simulink model "sl_EstimacDinamic"  (Simulink 9.1)
settings: Solver=ode45  StartTime=0.0  StopTime=40  RelTol=1e-8  EnableMultiTasking=on
values from neighbouring files (symbols this model uses):
  Aa_1 = Aa_1/50    (= 0.004)    [DatosSimAcDir_Exp.m]    (also in DatosSimSenoides.m = 1; DatosSimSenoides_Exp.m = 2)
  Aa_2 = Aa_2/30    (= 6.66666666667)    [DatosSimAcDir_Exp.m]    (also in DatosSimSenoides.m = 1; DatosSimSenoides_Exp.m = 0.5)
  Aa_3 = Aa_3/15    (= 0.266666666667)    [DatosSimAcDir_Exp.m]    (also in DatosSimSenoides.m = 5; DatosSimSenoides_Exp.m = 0.5)
  Ab_1 = Ab_1/50    (= 6e-05)    [DatosSimAcDir_Exp.m]    (also in DatosSimSenoides.m = 2; DatosSimSenoides_Exp.m = 3)
  Ab_3 = Ab_3/15    (= 1)    [DatosSimAcDir_Exp.m]    (also in DatosSimSenoides.m = 6; DatosSimSenoides_Exp.m = 2)
  Im_cc1 = Im_cc1/50    (= 0)    [DatosSimAcDir_Exp.m]    (also in DatosSimSenoides.m; DatosSimSenoides_Exp.m)
  Im_cc2 = Im_cc2/30    (= 96.6666666667)    [DatosSimAcDir_Exp.m]    (also in DatosSimSenoides.m = 0; DatosSimSenoides_Exp.m = 14)
  Im_cc3 = Im_cc3/15    (= 1)    [DatosSimAcDir_Exp.m]    (also in DatosSimSenoides.m = 0; DatosSimSenoides_Exp.m = 3)
  tau1 = 1    [DatosSimAcDir_Exp.m]    (also in DatosSimSenoides.m = 5; DatosSimSenoides_Exp.m = 0.01)
  Tm = 0.001    [AnalisisFrecuencial.m]    (also in ComparativaModelo.m; DatosSimSenoides.m = 0.01; GDT_C_RRR.m; controlador.m)
  wa_1 = 10    [DatosSimAcDir_Exp.m]    (also in DatosSimSenoides.m = 0.5; DatosSimSenoides_Exp.m)
  wa_2 = 40    [DatosSimAcDir_Exp.m]    (also in DatosSimSenoides.m = 3; DatosSimSenoides_Exp.m = 15)
  wa_3 = 8    [DatosSimAcDir_Exp.m]    (also in DatosSimSenoides.m = 0.5; DatosSimSenoides_Exp.m)
  wb_1 = 3    [DatosSimAcDir_Exp.m]    (also in DatosSimSenoides.m = 1; DatosSimSenoides_Exp.m)
  wb_3 = 50    [DatosSimAcDir_Exp.m]    (also in DatosSimSenoides.m = 1; DatosSimSenoides_Exp.m = 3)
libraries: simulink x1
settings Model: Creator=Manuel G. Ortega  LastModifiedBy=MAMG  ExtModeTrigMode=oneshot  ExtModeArmWhenConnect=off
settings DataIOCC: SignalLoggingSaveFormat=ModelDataLogs
settings OptimizationCC: BooleanDataType=off  ExpressionDepthLimit=2147483647  InitFltsAndDblsToZero=on
settings DebuggingCC: SaveWithParameterizedLinksMsg=none  SignalResolutionControl=TryResolveAllWithWarning  MultiTaskDSMMsg=warning  MultiTaskCondExecSysMsg=none  FcnCallInpInsideContextMsg=warning  StateNameClashWarn=warning
settings HardwareCC: TargetUnknown=on
settings GRTTargetCC: TargetFcnLib=ansi_tfl_tmw.mat  GeneratePreprocessorConditionals=Disable all
settings ConfigComp: CovSFcnEnable=off

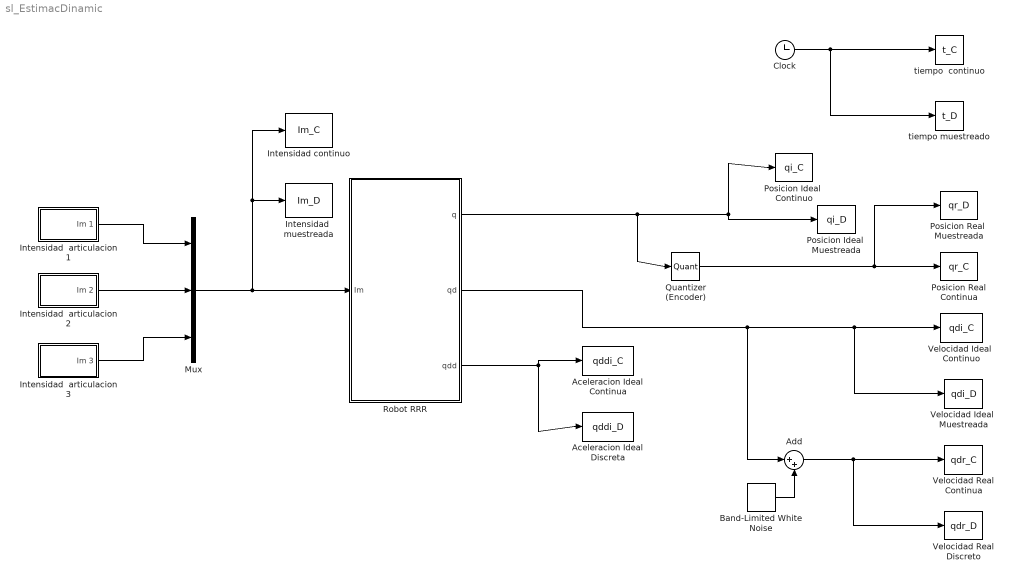
== system sl_EstimacDinamic ==
  Aceleracion Ideal Continua : ToWorkspace  VariableName=qddi_C  SampleTime=-1
  Aceleracion Ideal Discreta : ToWorkspace  VariableName=qddi_D  SampleTime=Tm
  Add : Sum  Inputs=|++
  Band-Limited White Noise : simulink/Sources/Band-Limited White Noise  Cov=[0.1]  Ts=0.1  seed=[23341]
  Clock : Clock
  Intensidad continuo : ToWorkspace  VariableName=Im_C  SampleTime=-1
  Intensidad  articulacion1 : Subsystem
  Intensidad  articulacion2 : Subsystem
  Intensidad  articulacion3 : Subsystem
  "Intensidad  muestreada " : ToWorkspace  VariableName=Im_D  SampleTime=Tm
  Mux : Mux  Inputs=3
  Posicion Ideal  Continuo : ToWorkspace  VariableName=qi_C  SampleTime=-1
  Posicion Ideal  Muestreada : ToWorkspace  VariableName=qi_D  SampleTime=Tm
  Posicion Real Continua : ToWorkspace  VariableName=qr_C  SampleTime=-1
  Posicion Real  Muestreada : ToWorkspace  VariableName=qr_D  SampleTime=Tm
  Quantizer (Encoder) : Quantizer
  Robot RRR : Subsystem
  Velocidad Ideal  Continuo : ToWorkspace  VariableName=qdi_C  SampleTime=-1
  Velocidad Ideal  Muestreada : ToWorkspace  VariableName=qdi_D  SampleTime=Tm
  Velocidad Real Continua : ToWorkspace  VariableName=qdr_C  SampleTime=-1
  Velocidad Real Discreto : ToWorkspace  VariableName=qdr_D  SampleTime=Tm
  tiempo muestreado : ToWorkspace  VariableName=t_D  SampleTime=Tm
  tiempo  continuo : ToWorkspace  VariableName=t_C  SampleTime=-1
  wires:
  Robot RRR/1(q) -> Quantizer (Encoder)/1, Posicion Ideal  Continuo/1, Posicion Ideal  Muestreada/1
  Robot RRR/3(qdd) -> Aceleracion Ideal Discreta/1, Aceleracion Ideal Continua/1
  Clock/1 -> tiempo  continuo/1, tiempo muestreado/1
  Mux/1 -> "Intensidad  muestreada "/1, Intensidad continuo/1, Robot RRR/1(Im)
  Quantizer (Encoder)/1 -> Posicion Real  Muestreada/1, Posicion Real Continua/1
  Robot RRR/2(qd) -> Add/1, Velocidad Ideal  Muestreada/1, Velocidad Ideal  Continuo/1
  Band-Limited White Noise/1 -> Add/2
  Add/1 -> Velocidad Real Continua/1, Velocidad Real Discreto/1
  Intensidad  articulacion1/1(Im 1) -> Mux/1
  Intensidad  articulacion3/1(Im 3) -> Mux/3
  Intensidad  articulacion2/1(Im 2) -> Mux/2

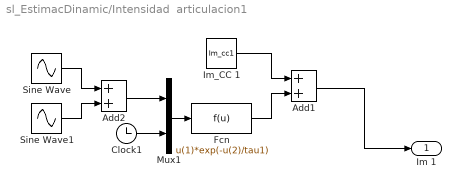
== system sl_EstimacDinamic/Intensidad  articulacion1 ==
  Add1 : Sum
  Add2 : Sum
  Clock1 : Clock
  Fcn : Fcn  Expr=u(1)*exp(-u(2)/tau1)
  "Im_CC 1 " : Constant  Value=Im_cc1
  Mux1 : Mux  Inputs=2
  Sine Wave : Sin  Amplitude=Aa_1  Frequency=wa_1  SampleTime=0
  Sine Wave1 : Sin  Amplitude=Ab_1  Frequency=wb_1  SampleTime=0
  Im 1 : Outport
  wires:
  Add2/1 -> Mux1/1
  "Im_CC 1 "/1 -> Add1/1
  Fcn/1 -> Add1/2
  Clock1/1 -> Mux1/2
  Add1/1 -> Im 1/1
  Mux1/1 -> Fcn/1
  Sine Wave1/1 -> Add2/2
  Sine Wave/1 -> Add2/1

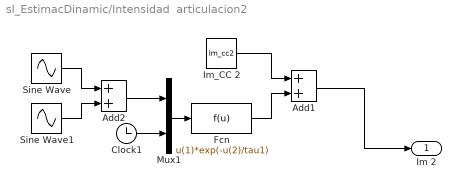
== system sl_EstimacDinamic/Intensidad  articulacion2 ==
  Add1 : Sum
  Add2 : Sum
  Clock1 : Clock
  Fcn : Fcn  Expr=u(1)*exp(-u(2)/tau1)
  "Im_CC 2 " : Constant  Value=Im_cc2
  Mux1 : Mux  Inputs=2
  Sine Wave : Sin  Amplitude=Aa_2  Frequency=wa_2  SampleTime=0
  Sine Wave1 : Sin  Amplitude=Ab_1  Frequency=wb_1  SampleTime=0
  Im 2 : Outport
  wires:
  Add2/1 -> Mux1/1
  "Im_CC 2 "/1 -> Add1/1
  Fcn/1 -> Add1/2
  Clock1/1 -> Mux1/2
  Add1/1 -> Im 2/1
  Mux1/1 -> Fcn/1
  Sine Wave1/1 -> Add2/2
  Sine Wave/1 -> Add2/1

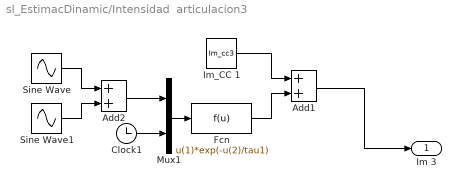
== system sl_EstimacDinamic/Intensidad  articulacion3 ==
  Add1 : Sum
  Add2 : Sum
  Clock1 : Clock
  Fcn : Fcn  Expr=u(1)*exp(-u(2)/tau1)
  "Im_CC 1 " : Constant  Value=Im_cc3
  Mux1 : Mux  Inputs=2
  Sine Wave : Sin  Amplitude=Aa_3  Frequency=wa_3  SampleTime=0
  Sine Wave1 : Sin  Amplitude=Ab_3  Frequency=wb_3  SampleTime=0
  Im 3 : Outport
  wires:
  Add2/1 -> Mux1/1
  "Im_CC 1 "/1 -> Add1/1
  Fcn/1 -> Add1/2
  Clock1/1 -> Mux1/2
  Add1/1 -> Im 3/1
  Mux1/1 -> Fcn/1
  Sine Wave1/1 -> Add2/2
  Sine Wave/1 -> Add2/1

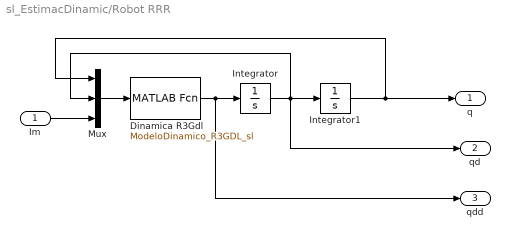
== system sl_EstimacDinamic/Robot RRR ==
  Im : Inport
  Dinamica R3Gdl : MATLABFcn  MATLABFcn=ModeloDinamico_R3GDL_sl  OutputDimensions=3
  Integrator : Integrator  InitialCondition=[0;0;0];
  Integrator1 : Integrator  InitialCondition=[0;0;0]
  Mux : Mux  Inputs=3
  q : Outport
  qd : Outport  Port=2
  qdd : Outport  Port=3
  wires:
  Mux/1 -> Dinamica R3Gdl/1
  Dinamica R3Gdl/1 -> Integrator/1, qdd/1
  Integrator/1 -> Integrator1/1, qd/1, Mux/2
  Integrator1/1 -> q/1, Mux/1
  Im/1 -> Mux/3
